simulink model "MPC_MPC_GivenPathTracking"  (Simulink 8.2)
settings: Solver=ode45  StartTime=0.0  StopTime=40  FixedStep=0.01  RelTol=1e-3
libraries: Solver_SF x1
settings Model: Creator=xuwei  LastModifiedBy=leoking99

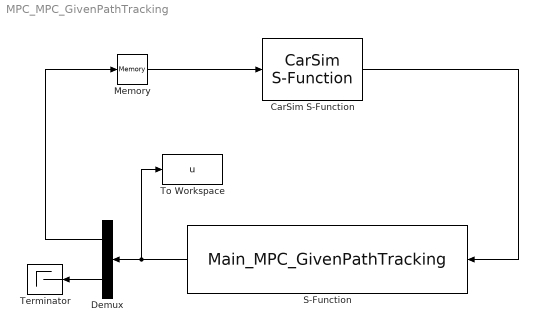
== system MPC_MPC_GivenPathTracking ==
  CarSim S-Function : Solver_SF/CarSim S-Function  Priority=1  VehicleCode=i_s  SIMFILE=LEO_MPC_GivenPathTrackingCtrl.sim
  Demux : Demux  Outputs=[2 7]
  Memory : Memory  X0=1  InheritSampleTime=on
  S-Function : S-Function  FunctionName=Main_MPC_GivenPathTracking  EnableBusSupport=off
  Terminator : Terminator
  To Workspace : ToWorkspace  VariableName=u  SampleTime=-1  SaveFormat=Structure
  wires:
  CarSim S-Function/1 -> S-Function/1
  S-Function/1 -> Demux/1, To Workspace/1
  Demux/2 -> Terminator/1
  Demux/1 -> Memory/1
  Memory/1 -> CarSim S-Function/1
